simulink model "simu"  (R2022b)
settings: Solver=VariableStepAuto  StartTime=0.0  StopTime=10.0  RelTol=1e-3
values from neighbouring files (symbols this model uses):
  A = zeros(taille_A)    [matrice.m]
undefined symbols (not defined in the file or in its folder): ans
libraries: simulink x1
settings Model: Creator=theog  LastModifiedBy=theog
settings ModelReferenceCC: EnableRefExpFcnMdlSchedulingChecks=on

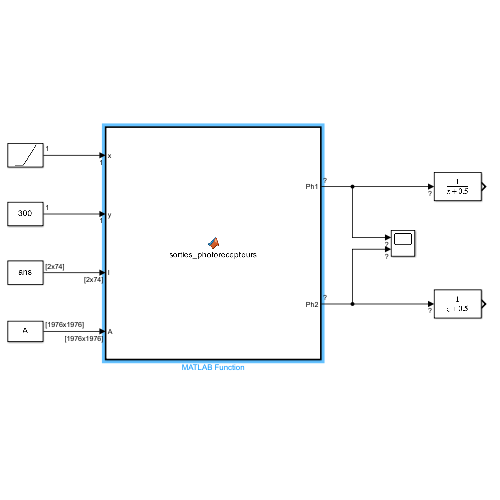
[thumbnail: Simulink's stored preview of the top-level diagram]
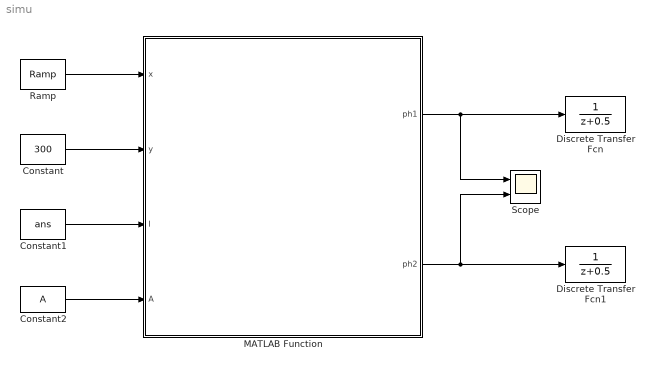
== system simu ==
  Constant : Constant  Value=300
  Constant1 : Constant  Value=ans
  Constant2 : Constant  Value=A
  Discrete Transfer Fcn : DiscreteTransferFcn
  Discrete Transfer Fcn1 : DiscreteTransferFcn
  MATLAB Function : MATLAB Function  TreatAsAtomicUnit=on
  Ramp : simulink/Sources/Ramp  slope=500  start=0  InitialOutput=0
  Scope : Scope  NumInputPorts=2
  wires:
  Constant1/1 -> MATLAB Function/3(I)
  Constant2/1 -> MATLAB Function/4(A)
  Constant/1 -> MATLAB Function/2(y)
  Ramp/1 -> MATLAB Function/1(x)
  MATLAB Function/1(ph1) -> Discrete Transfer Fcn/1, Scope/1
  MATLAB Function/2(ph2) -> Discrete Transfer Fcn1/1, Scope/2

== matlab function simu/MATLAB Function ==
  data: x input; ph1 output; y input; I input; ph2 output; A input
function [ph1,ph2]=sorties_photorecepteurs(x,y,I,A)
% importation du tableau d'environnement
%I = bandes;
%x = 500;
%y = 1000;
[~,nb_bandes]=size(I);
xn = I(1,:);
In = I(2,:);
deltarho=3.8;
thetamax = 2.6*deltarho;
% création du tableau contenant les angles
theta=zeros(1,nb_bandes);
for i=1:nb_bandes
    theta(i)=rad2deg(atan2(-y,xn(i)-x));
end

%réduction du tableau aux champs perçus par les deux photorécepteurs,
%respectivement :

%photorécepteur 1
index1a= -90 - (1.3*deltarho) - (deltarho/2);
index1b= -90 - (deltarho/2) + (1.3*deltarho);
idxchamp=find((theta>=index1a)&(theta<=index1b));
theta1 = theta(idxchamp);
[~,taille1] = size(theta1);
%reacalibration numérique 1
for i=1:taille1
    theta1(i) = abs(theta1(i)+90+(deltarho/2)+(1.3*deltarho))/thetamax*1976;
end
%calcul final pour ph1
ph1=0;
if taille1>1
    for i=1:taille1-1
        if(i==1)
            ph1 = ph1+ In(idxchamp(i))*A(ceil(theta1(i)),1);
        elseif(i==taille1-1)
            ph1 = ph1+ In(idxchamp(i))*A(1976,ceil(theta1(i)));
        else
            ph1 = ph1 + In(idxchamp(i))*A(ceil(theta1(i+1)),ceil(theta1(i)));
        end
    end
elseif taille1==1
     ph1 = ph1+ In(idxchamp(1))*A(ceil(theta1(1)),1);
     ph1 = ph1+ In(idxchamp(1))*A(1976,ceil(theta1(1)));
else
    ph1 = 0;
end

%photorecepteur 2
index2a= -90 - (1.3*deltarho) + (deltarho/2);
index2b= -90 + (deltarho/2) + (1.3*deltarho);

idxchamp2=find((theta>=index2a)&(theta<=index2b));
theta2 = theta(idxchamp2);
[~,taille2]=size(theta2);

%reacalibration numérique 2
for i=1:taille2
    theta2(i) = abs(theta2(i)+90-(deltarho/2)+(1.3*deltarho))/thetamax*1976;
end

%calcul final pour ph2
ph2=0;
if taille2>1
    for i=1:taille2-1
        if(i==1)
            ph2= ph2+ In(idxchamp2(i))*A(ceil(theta2(i)),1);
        elseif(i==taille2-1)
            ph2 = ph2+ In(idxchamp2(i))*A(1976,ceil(theta2(i)));
        else
            ph2 = ph2 + In(idxchamp2(i))*A(ceil(theta2(i+1)),ceil(theta2(i)));
        end
    end
elseif taille2==1
     ph2 = ph2+ In(idxchamp2(1))*A(ceil(theta2(1)),1);
     ph2 = ph2+ In(idxchamp2(1))*A(1976,ceil(theta2(1)));
else
    ph2 = 0;
end
end
